simulink model "PendulumPositionControl_PD"  (R2020b)
settings: Solver=VariableStepAuto  StartTime=0.0  StopTime=10.0  RelTol=1e-3  EnableMultiTasking=on
values from neighbouring files (symbols this model uses):
  b = 4.425*1e-6    (= 4.425e-06)    [PendulumRotorPositionControl.m]    (also in rotor10Hz.m; rotor10Hz_aruul.m)
  J_pend = J_rotor    (= 1.8053e-05)    [PendulumRotorPositionControl.m]    (also in rotor10Hz.m; rotor10Hz_aruul.m)
  K_g = m*g*l_c    (= 0.0080536176)    [PendulumRotorPositionControl.m]    (also in rotor10Hz.m; rotor10Hz_aruul.m)
  K_m = 0.025463    [PendulumRotorPositionControl.m]    (also in rotor10Hz.m; rotor10Hz_aruul.m)
  K_pend = 0    [PendulumRotorPositionControl.m]    (also in rotor10Hz.m; rotor10Hz_aruul.m)
  K_sin = cos(Angle_Pendu)    [PendulumRotorPositionControl.m]    (also in rotor10Hz.m; rotor10Hz_aruul.m)
  L = 0    [PendulumRotorPositionControl.m]    (also in rotor10Hz.m; rotor10Hz_aruul.m)
  R = 6    [PendulumRotorPositionControl.m]    (also in rotor10Hz.m; rotor10Hz_aruul.m)
  saturation = 1.0    (= 1)    [PendulumRotorPositionControl.m]    (also in rotor10Hz.m; rotor10Hz_aruul.m)
  Tcomp = 0.0005*Ts*14    (= 0.0007)    [PendulumRotorPositionControl.m]    (also in rotor10Hz.m; rotor10Hz_aruul.m)
  Ts = 0.1    [PendulumRotorPositionControl.m]    (also in rotor10Hz.m; rotor10Hz_aruul.m)
  Tss = 1/20000    (= 5e-05)    [PendulumRotorPositionControl.m]    (also in rotor10Hz.m; rotor10Hz_aruul.m)
  V_s = 10.5    [PendulumRotorPositionControl.m]    (also in rotor10Hz.m; rotor10Hz_aruul.m)
undefined symbols (not defined in the file or in its folder): C_den, C_num
libraries: simulink x1
settings Model: Creator=Martin  LastModifiedBy=TC Tsao
settings SolverCC: ZeroCrossControl=DisableAll  ZeroCrossAlgorithm=Adaptive
settings DataIOCC: ReturnWorkspaceOutputs=off
settings OptimizationCC: LifeSpan=inf
settings DebuggingCC: MaxConsecutiveZCsMsg=none  SFUnexpectedBacktrackingDiag=warning  SFNoUnconditionalDefaultTransitionDiag=warning  SFExecutionAtInitializationDiag=none  ArithmeticOperatorsInVariantConditions=warning
settings SFSimCC: SimUseLocalCustomCode=off  CustomCodeUndefinedFunction=UseInterfaceOnly
settings RTWCC: RTWUseLocalCustomCode=off
settings CodeAppCC: StateflowObjectComments=on
settings GRTTargetCC: TargetLangStandard=C89/C90 (ANSI)
settings ConfigComp: CovMetricSettings=dw  CovSaveCumulativeToWorkspaceVar=on  CovSaveSingleToWorkspaceVar=on  CovExternalEMLEnable=off

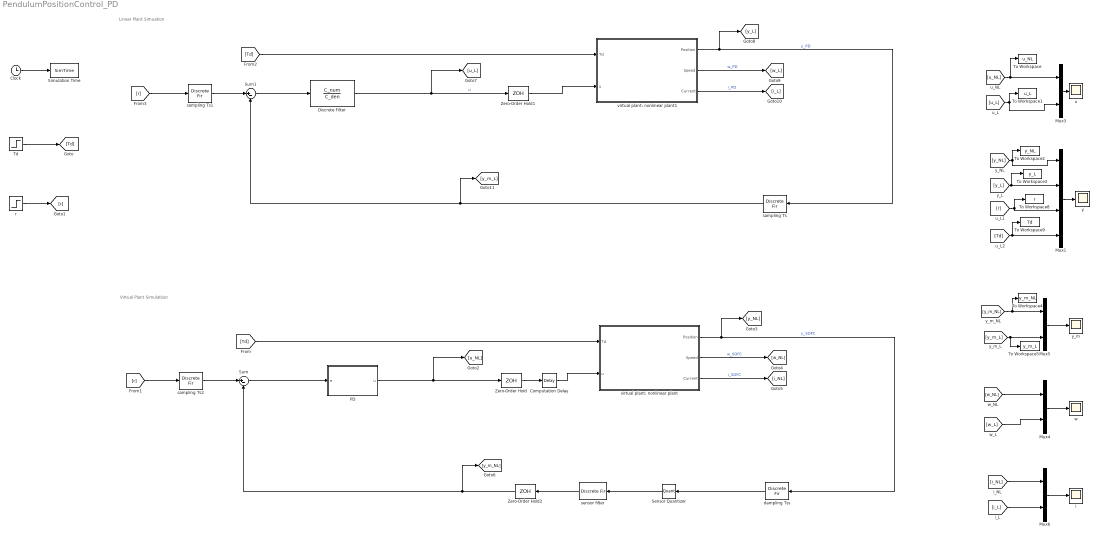
== system PendulumPositionControl_PD ==
  note: Linear Plant Simuation
  note: Virtual Plant Simulatiion
  Clock : Clock
  Computation Delay : TransportDelay  DelayTime=Tcomp  BufferSize=4096  PadeOrder=2
  Discrete Filter : DiscreteFilter  Numerator=C_num  Denominator=C_den  InputProcessing=Columns as channels (frame based)
  Mux1 : Mux
  Mux{3..6} (4 alike) : Mux  Inputs=2
  PD : MATLAB Function  TreatAsAtomicUnit=on  mask{Numerator=C_num, Denomenator=C_den}
  Sensor Quantizer : Quantizer  QuantizationInterval=encoder_resolution
  Simulation Time : ToWorkspace  VariableName=SimTime  SampleTime=-1
  Sum : Sum  Inputs=|+-
  Sum1 : Sum  Inputs=|+-
  Td : Step  Time=5  After=0.05  SampleTime=0
  To Workspace : ToWorkspace  VariableName=u_NL  SampleTime=Ts
  To Workspace1 : ToWorkspace  VariableName=u_L  SampleTime=Ts
  To Workspace2 : ToWorkspace  VariableName=y_NL  SampleTime=Ts
  To Workspace3 : ToWorkspace  VariableName=y_L  SampleTime=Ts
  To Workspace4 : ToWorkspace  VariableName=y_m_NL  SampleTime=Ts
  To Workspace5 : ToWorkspace  VariableName=y_m_L  SampleTime=Ts
  To Workspace8 : ToWorkspace  VariableName=r  SampleTime=Ts
  To Workspace9 : ToWorkspace  VariableName=Td  SampleTime=Ts
  Zero-Order Hold : ZeroOrderHold  SampleTime=Ts
  Zero-Order Hold1 : ZeroOrderHold  SampleTime=Ts
  Zero-Order Hold2 : ZeroOrderHold  SampleTime=Ts
  dampling Tss : DiscreteFir  Coefficients=[1]  SampleTime=Tss
  i : Scope
  r : Step  SampleTime=Ts
  sampling Ts : DiscreteFir  Coefficients=[1]  SampleTime=Ts
  sampling Ts1 : DiscreteFir  Coefficients=[1]  SampleTime=Ts
  sampling Ts2 : DiscreteFir  Coefficients=[1]  SampleTime=Ts
  sensor filter : DiscreteFir  Coefficients=[0.25 0.25 0.25 0.25]
  u : Scope
  virtual plant: nonlinear plant : Subsystem
  virtual plant: nonlinear plant1 : Subsystem
  "w\t" : Scope
  y : Scope
  y_m : Scope
  wires:
  Clock/1 -> Simulation Time/1
  virtual plant: nonlinear plant/1(Position) -> [y_NL], dampling Tss/1  "y_SOFC"
  virtual plant: nonlinear plant/2(Speed) -> [w_NL]  "w_SOFC"
  virtual plant: nonlinear plant/3(Current) -> [i_NL]  "i_SOFC"
  Sensor Quantizer/1 -> sensor filter/1
  dampling Tss/1 -> Sensor Quantizer/1
  Zero-Order Hold/1 -> Computation Delay/1
  Td/1 -> [Td]
  r/1 -> [r]
  [Td] -> virtual plant: nonlinear plant/1(Td)
  sensor filter/1 -> Zero-Order Hold2/1
  Sum/1 -> PD/1(e)
  Zero-Order Hold2/1 -> Sum/2, [y_m_NL]
  [u_NL] -> To Workspace/1, Mux3/1
  Mux3/1 -> u/1
  Mux1/1 -> y/1
  [y_NL] -> To Workspace2/1, Mux1/1
  [y_L] -> To Workspace3/1, Mux1/2
  Mux5/1 -> y_m/1
  [y_m_NL] -> To Workspace4/1, Mux5/1
  [y_m_L] -> To Workspace5/1, Mux5/2
  PD/1(u) -> [u_NL], Zero-Order Hold/1
  Mux4/1 -> "w\t"/1
  [w_NL] -> Mux4/1
  [w_L] -> Mux4/2
  Mux6/1 -> i/1
  [i_NL] -> Mux6/1
  [i_L] -> Mux6/2
  Discrete Filter/1 -> [u_L], Zero-Order Hold1/1  "u"
  virtual plant: nonlinear plant1/1(Position) -> [y_L], sampling Ts/1  "y_PD"
  virtual plant: nonlinear plant1/3(Current) -> [i_L]  "i_PD"
  sampling Ts/1 -> Sum1/2, [y_m_L]
  virtual plant: nonlinear plant1/2(Speed) -> [w_L]  "w_PD"
  Zero-Order Hold1/1 -> virtual plant: nonlinear plant1/2(u)
  Sum1/1 -> Discrete Filter/1
  [u_L] -> To Workspace1/1, Mux3/2
  Computation Delay/1 -> virtual plant: nonlinear plant/2(u)
  [r] -> sampling Ts1/1
  [Td] -> virtual plant: nonlinear plant1/1(Td)
  [r] -> sampling Ts2/1
  [r] -> To Workspace8/1, Mux1/3
  [Td] -> Mux1/4, To Workspace9/1
  sampling Ts1/1 -> Sum1/1
  sampling Ts2/1 -> Sum/1

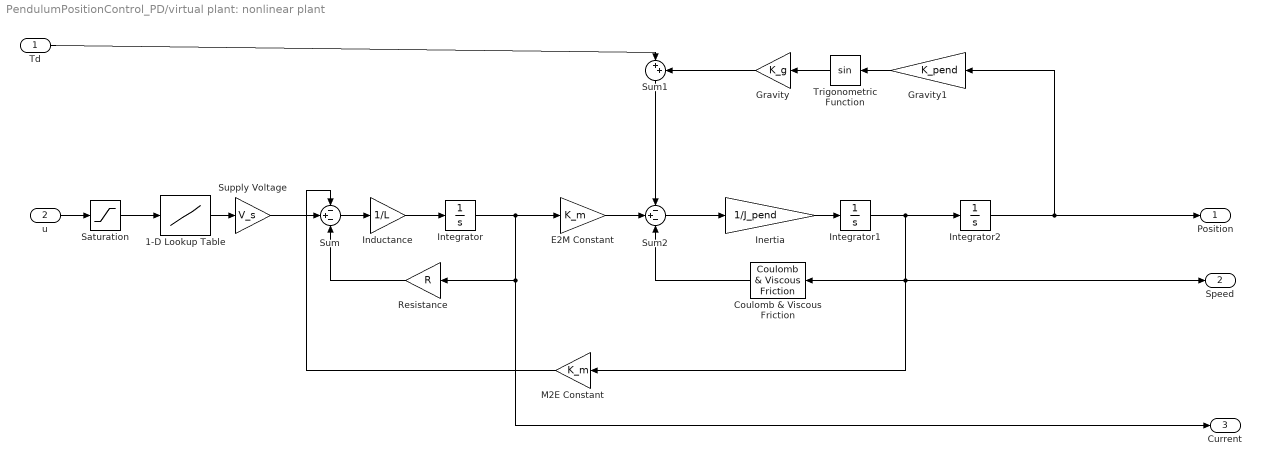
== system PendulumPositionControl_PD/virtual plant: nonlinear plant ==
  Td : Inport
  u : Inport  Port=2
  1-D Lookup Table : Lookup_n-D  NumberOfTableDimensions=1  BreakpointsForDimension1=[-1,-0.96,-0.1,-0.06,-0.04,0,0.04,0.06,0.1,0.96,1]  Table=[-10.8,-10.8,-2,-1,-0,0,0,1,2,10.8,10.8]/V_s  InternalRulePriority=Speed  RndMeth=Simplest  InputSameDT=on
  Coulomb & Viscous Friction : simulink/Discontinuities/Coulomb & Viscous Friction  offset=Friction_static  gain=b
  E2M Constant : Gain  Gain=K_m
  Gravity : Gain  Gain=K_g
  Gravity1 : Gain  Gain=K_pend
  Inductance : Gain  Gain=1/L
  Inertia : Gain  Gain=1/J_pend
  Integrator : Integrator
  Integrator1 : Integrator
  Integrator2 : Integrator
  M2E Constant : Gain  Gain=K_m
  Resistance : Gain  Gain=R
  Saturation : Saturate  UpperLimit=saturation  LowerLimit=-saturation
  Sum : Sum  Inputs=-+-
  Sum1 : Sum  Inputs=|++
  Sum2 : Sum  Inputs=-+-
  Supply Voltage : Gain  Gain=V_s
  Trigonometric Function : Trigonometry
  Position : Outport
  Speed : Outport  Port=2
  Current : Outport  Port=3
  wires:
  Coulomb & Viscous Friction/1 -> Sum2/3
  Gravity/1 -> Sum1/2
  Integrator/1 -> E2M Constant/1, Current/1, Resistance/1
  Integrator1/1 -> Coulomb & Viscous Friction/1, Speed/1, M2E Constant/1, Integrator2/1
  Resistance/1 -> Sum/3
  Trigonometric Function/1 -> Gravity/1
  Sum/1 -> Inductance/1
  Inductance/1 -> Integrator/1
  Supply Voltage/1 -> Sum/2
  M2E Constant/1 -> Sum/1
  Sum2/1 -> Inertia/1
  Inertia/1 -> Integrator1/1
  Saturation/1 -> 1-D Lookup Table/1
  u/1 -> Saturation/1
  E2M Constant/1 -> Sum2/2
  Integrator2/1 -> Position/1, Gravity1/1
  1-D Lookup Table/1 -> Supply Voltage/1
  Td/1 -> Sum1/1
  Gravity1/1 -> Trigonometric Function/1
  Sum1/1 -> Sum2/1

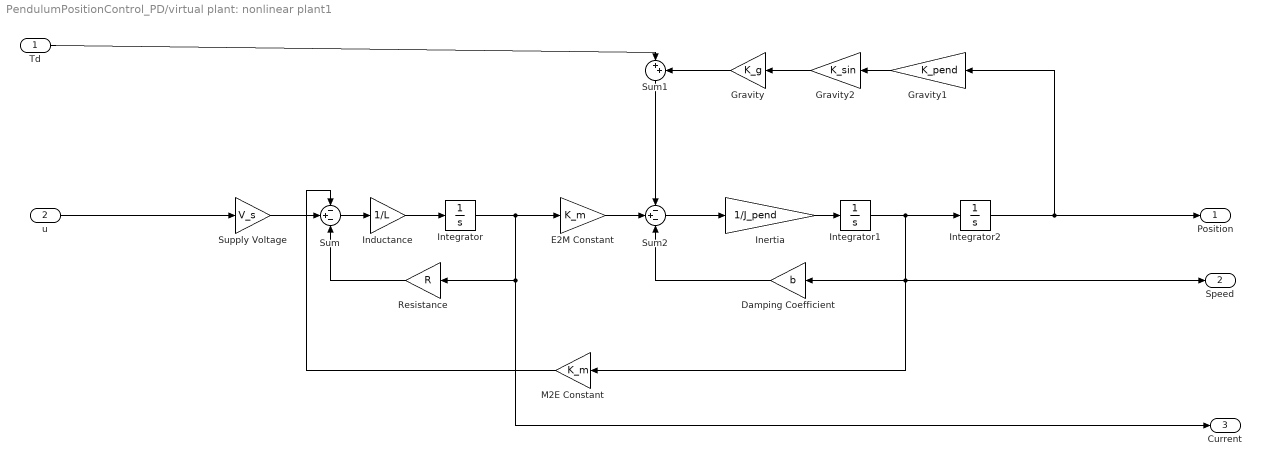
== system PendulumPositionControl_PD/virtual plant: nonlinear plant1 ==
  Td : Inport
  u : Inport  Port=2
  Damping Coefficient : Gain  Gain=b
  E2M Constant : Gain  Gain=K_m
  Gravity : Gain  Gain=K_g
  Gravity1 : Gain  Gain=K_pend
  Gravity2 : Gain  Gain=K_sin
  Inductance : Gain  Gain=1/L
  Inertia : Gain  Gain=1/J_pend
  Integrator : Integrator
  Integrator1 : Integrator
  Integrator2 : Integrator
  M2E Constant : Gain  Gain=K_m
  Resistance : Gain  Gain=R
  Sum : Sum  Inputs=-+-
  Sum1 : Sum  Inputs=|++
  Sum2 : Sum  Inputs=-+-
  Supply Voltage : Gain  Gain=V_s
  Position : Outport
  Speed : Outport  Port=2
  Current : Outport  Port=3
  wires:
  Damping Coefficient/1 -> Sum2/3
  Gravity/1 -> Sum1/2
  Integrator/1 -> E2M Constant/1, Current/1, Resistance/1
  Integrator1/1 -> Speed/1, M2E Constant/1, Damping Coefficient/1, Integrator2/1
  Resistance/1 -> Sum/3
  Gravity2/1 -> Gravity/1
  Sum/1 -> Inductance/1
  Inductance/1 -> Integrator/1
  Supply Voltage/1 -> Sum/2
  M2E Constant/1 -> Sum/1
  Sum2/1 -> Inertia/1
  Inertia/1 -> Integrator1/1
  E2M Constant/1 -> Sum2/2
  Integrator2/1 -> Position/1, Gravity1/1
  u/1 -> Supply Voltage/1
  Td/1 -> Sum1/1
  Gravity1/1 -> Gravity2/1
  Sum1/1 -> Sum2/1

== matlab function PendulumPositionControl_PD/PD ==
  data: e input; u output; Numerator parameter; Denomenator parameter

function u = controller(e,Numerator, Denomenator)
a0=Denomenator(1);
a1=Denomenator(2)/a0;

b0=Numerator(1)/a0;
b1= Numerator(2)/a0;

persistent u_update;
  if isempty(u_update)  %local variable initialization
        u_update=0;   
  end


%Transfer function C(z)= (b0z^2+b1z)/(z^2+a1z)=(b0+b1z^-1)/(1+a1z^-1)
% 
%Difference equation u(k)= -a1*u(k-1)+ b0*e(k)+b1*e(k-1)
%Real time coding (correct):  
% u(k)= -a1*u(k-1)+ b0*e(k)+b1*e(k-1)=u_update + b0*e
u = u_update + b0*e ; %estimation (for current step update) (3 CPU operations)
% Send the control out to DAC here to minimize computation delay 
% DAC_out = u
         %prediction (for next step update)
         % u(k+1)= -a1*u(k)+ b0*e(k+1)+b1*e(k)= u_update + b0*e
         % u_update = -a1*u+b1*e
u_update=-a1*u+b1*e;  %(7 CPU OPs after sending out DAC)

%Real time coding (incorrect): 
%u = -a1*u1 + b1*e1 + b0*e ; % (7 CPU OPs)
%         u1=u;
%         e1=e;  %(2 CPU Ops)
% Sending the control out to DAC here at end of computation renders computation delay 
%(9 CPU OPs)
% DAC_out = u
